simulink model "WT_Gearbox_AV"  (R2020a)
settings: Solver=ode23t  StartTime=0.0  StopTime=10.0  RelTol=1e-3
libraries: fl_lib x20, nesl_utility x5, sdl_lib x3
settings Model: Creator=Jayan Joshua  LastModifiedBy=Jayan Joshua

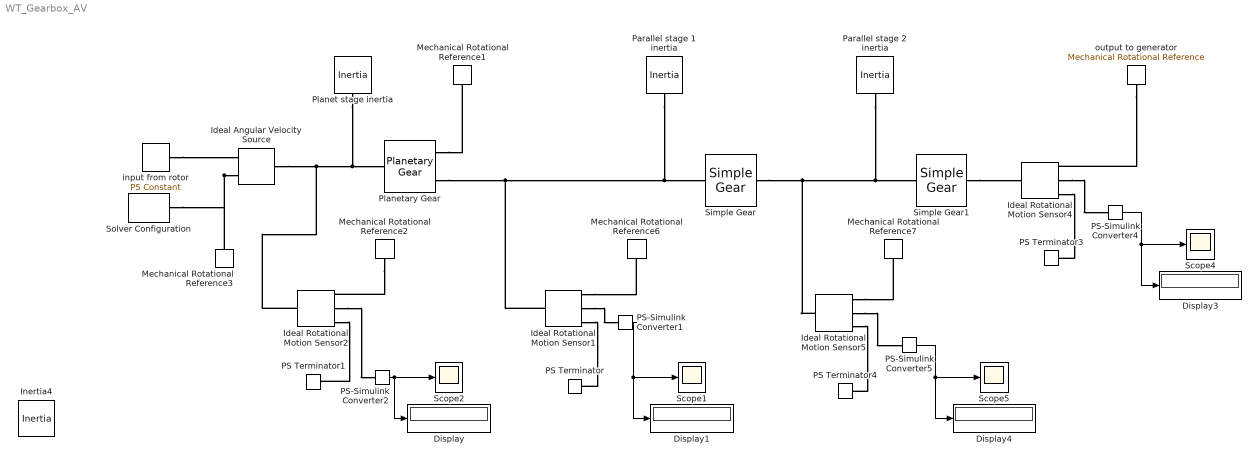
== system WT_Gearbox_AV ==
  Display{,1,3..4} (4 alike) : Display
  Ideal Angular Velocity Source : fl_lib/Mechanical/Mechanical Sources/Ideal Angular Velocity Source
  Ideal Rotational Motion Sensor{1..2,4..5} (4 alike) : fl_lib/Mechanical/Mechanical Sensors/Ideal Rotational Motion Sensor  wrap_angle=simscape.enum.onoff.off  offset=0 rad
  Inertia4 : fl_lib/Mechanical/Rotational Elements/Inertia  inertia=1000 kg*m^2  w_specify=off  w_priority=High  w=0 rad/s  w_nominal_specify=off  w_nominal_unit=rad/s  w_nominal_value=1  t_specify=off  t_priority=None  t=0 N*m  t_nominal_specify=off  t_nominal_unit=N*m  t_nominal_value=1
  Mechanical Rotational Reference{1..3,6..7} (5 alike) : fl_lib/Mechanical/Rotational Elements/Mechanical Rotational Reference
  PS Terminator{,1,3..4} (4 alike) : fl_lib/Physical Signals/Sinks/PS Terminator
  PS-Simulink Converter{1..2,4..5} (4 alike) : nesl_utility/PS-Simulink Converter  PhysicalDomain=network_engine_domain  SubClassName=ps_output  LeftPortType=input  RightPortType=output  PseudoPeriodic=off  Frequencies=[]  Unit=inherit  AffineConversion=off
  Parallel stage 1 inertia : fl_lib/Mechanical/Rotational Elements/Inertia  inertia=100 kg*m^2  w_specify=off  w_priority=High  w=0 rad/s  w_nominal_specify=off  w_nominal_unit=rad/s  w_nominal_value=1  t_specify=off  t_priority=None  t=0 N*m  t_nominal_specify=off  t_nominal_unit=N*m  t_nominal_value=1
  Parallel stage 2 inertia : fl_lib/Mechanical/Rotational Elements/Inertia  inertia=100 kg*m^2  w_specify=off  w_priority=High  w=0 rad/s  w_nominal_specify=off  w_nominal_unit=rad/s  w_nominal_value=1  t_specify=off  t_priority=None  t=0 N*m  t_nominal_specify=off  t_nominal_unit=N*m  t_nominal_value=1
  Planet stage inertia : fl_lib/Mechanical/Rotational Elements/Inertia  inertia=100 kg*m^2  w_specify=off  w_priority=High  w=0 rad/s  w_nominal_specify=off  w_nominal_unit=rad/s  w_nominal_value=1  t_specify=off  t_priority=None  t=0 N*m  t_nominal_specify=off  t_nominal_unit=N*m  t_nominal_value=1
  Planetary Gear : sdl_lib/Gears/Planetary Gear  rs_ratio=7  friction_model=sdl.enum.gear_friction.none  mu_visc=[0, 0] N*m/(rad/s)  efficiency=[.96, .98]  temperature_TLU=[280, 300, 320] K  efficiency_sp_TLU=[.95, .9, .85]  efficiency_rp_TLU=[.95, .9, .85]  pwr_thr=[.001, .001] W  thermal_mass=50 J/K  T_init=300 K  model_inertia=simscape.enum.onoff.off  planet_inertia=100 kg*m^2
      settings: SourceProductBaseCode=LD
  Scope{1..2,4..5} (4 alike) : Scope
  Simple Gear : sdl_lib/Gears/Simple Gear  ratio=1/4.5  rotation_direction=2  friction_model=sdl.enum.gear_efficiencies_load.off  T_noload=0.1 N*m  T_nom=5 N*m  efficiency_nom=0.8  efficiency=0.8  mu_visc=[0, 0] N*m/(rad/s)  w_thr=0.01 rad/s  pwr_thr=0.001 W  enable_faults=simscape.enum.onoff.off  efficiency_fault=0.05  external_fault=simscape.enum.onoff.off  temporal_fault=simscape.enum.onoff.off  fault_time=5 s  fault_angles=pi / 12 rad  report_fault=1  temperature_TLU=[280, 300, 320] K  load_TLU=[1, 5, 10] N*m  efficiency_TLU=[.95, .9, .85]  efficiency_TLU2=[.85, .8, .75; .95, .9, .85; .85, .8, .7]  thermal_mass=50 J/K  T_init=300 K
  Simple Gear1 : sdl_lib/Gears/Simple Gear  ratio=1/3.15  rotation_direction=2  friction_model=sdl.enum.gear_efficiencies_load.off  T_noload=0.1 N*m  T_nom=5 N*m  efficiency_nom=0.8  efficiency=0.8  mu_visc=[0, 0] N*m/(rad/s)  w_thr=0.01 rad/s  pwr_thr=0.001 W  enable_faults=simscape.enum.onoff.off  efficiency_fault=0.05  external_fault=simscape.enum.onoff.off  temporal_fault=simscape.enum.onoff.off  fault_time=5 s  fault_angles=pi / 12 rad  report_fault=1  temperature_TLU=[280, 300, 320] K  load_TLU=[1, 5, 10] N*m  efficiency_TLU=[.95, .9, .85]  efficiency_TLU2=[.85, .8, .75; .95, .9, .85; .85, .8, .7]  thermal_mass=50 J/K  T_init=300 K
  Solver Configuration : nesl_utility/Solver Configuration  PhysicalDomain=network_engine_domain  SubClassName=solver  LeftPortType=input  RightPortType=generic  Tones=[]  Harmonics=[]  SimulateNoise=off  Profile=off  UseLocalSampling=off  EnableSwitchedLinearOptims=on  FrequencyDomain=off  UseCCode=off  RelTol=0.001  AbsTol=1e-06  MinStep=1e-09  ToWorkspace=off  RevertToSquareIcSolve=off  NumHomotopyIterations=100  PhasorMode=off  PhasorModeNumHarmonics=1  DoDC=off  ResidualTolerance=1e-09  UseLocalSolver=off  LocalSolverChoice=NE_BACKWARD_EULER_ADVANCER  LocalSolverSampleTime=0.001  DoFixedCost=off  MaxNonlinIter=3  MaxModeIter=2  LinearAlgebra=auto  EquationFormulation=NE_TIME_EF  DelaysMemoryBudget=1024  AutomaticFiltering=on  FilteringTimeConstant=0.001  PartitionStorageMethod=AS_NEEDED  PartitionMemoryBudget=1024  PartitionMethod=ROBUST
  input from rotor : fl_lib/Physical Signals/Sources/PS Constant  constant=1.56 rad/s
  output to generator : fl_lib/Mechanical/Rotational Elements/Mechanical Rotational Reference
  wires:
  PS-Simulink Converter1/1 -> Scope1/1, Display1/1
  PS-Simulink Converter2/1 -> Display/1, Scope2/1
  PS-Simulink Converter4/1 -> Display3/1, Scope4/1
  PS-Simulink Converter5/1 -> Display4/1, Scope5/1
  connections:
  input from rotor/RConn1 -- Ideal Angular Velocity Source/RConn1
  Ideal Angular Velocity Source/RConn2 -- Mechanical Rotational Reference3/LConn1 -- Solver Configuration/RConn1
  Planetary Gear/RConn1 -- Mechanical Rotational Reference1/LConn1
  Ideal Rotational Motion Sensor1/RConn2 -- PS-Simulink Converter1/LConn1
  Mechanical Rotational Reference2/LConn1 -- Ideal Rotational Motion Sensor2/RConn1
  Ideal Rotational Motion Sensor2/RConn2 -- PS-Simulink Converter2/LConn1
  Ideal Rotational Motion Sensor1/RConn3 -- PS Terminator/LConn1
  Ideal Rotational Motion Sensor2/RConn3 -- PS Terminator1/LConn1
  Ideal Angular Velocity Source/LConn1 -- Ideal Rotational Motion Sensor2/LConn1 -- Planet stage inertia/LConn1 -- Planetary Gear/LConn1
  Simple Gear1/RConn1 -- Ideal Rotational Motion Sensor4/LConn1
  Ideal Rotational Motion Sensor4/RConn2 -- PS-Simulink Converter4/LConn1
  Ideal Rotational Motion Sensor4/RConn3 -- PS Terminator3/LConn1
  output to generator/LConn1 -- Ideal Rotational Motion Sensor4/RConn1
  Ideal Rotational Motion Sensor5/RConn2 -- PS-Simulink Converter5/LConn1
  Ideal Rotational Motion Sensor5/RConn3 -- PS Terminator4/LConn1
  Ideal Rotational Motion Sensor5/RConn1 -- Mechanical Rotational Reference7/LConn1
  Planetary Gear/RConn2 -- Ideal Rotational Motion Sensor1/LConn1 -- Simple Gear/LConn1 -- Parallel stage 1 inertia/LConn1
  Ideal Rotational Motion Sensor1/RConn1 -- Mechanical Rotational Reference6/LConn1
  Simple Gear/RConn1 -- Ideal Rotational Motion Sensor5/LConn1 -- Parallel stage 2 inertia/LConn1 -- Simple Gear1/LConn1
